simulink model "EVdemo_6"  (R2013b)
settings: Solver=FixedStepDiscrete  SolverMode=SingleTasking  StartTime=0.0  StopTime=650  FixedStep=4e-5  MaxStep=1e-5  RelTol=1e-3
InitFcn:
  | %EV_Param_Update
  | % update the number of strings (discretized)
  | numStrings = round(Opti_numStrings);
  | %disp(['Number of strings: ' num2str(numStrings)])
  | % update the effective capacity based on the number of strings
  | EV_Param.Battery_Det.Rated_Capacity = 28.5*numStrings; %A*hr
  | EV_Param.Battery_Det.DP = 1.5*fliplr([1500 1500 1600 1450 1325 1125 925 675 425 175 ])./8*EV_Param.Battery_Det.Rated_Capacity; % 8 comes from the 8Ahr rated batter data used (normalize and rescale to the rated capacity
  | EV_Param.Battery_Det.CP = fliplr([25 100 200 250 375 550 750 950 1125 1150])./8*EV_Param.Battery_Det.Rated_Capacity;
  | 
  | % update the number of cells in a string (discretized)
  | numSeriesCells = round(Opti_numSeriesCells);
  | %disp(['Number of cells in a string: ' num2str(numSeriesCells)])
  | % update the nominal string volage and charge deficit
  | EV_Param.Battery_Det.Nominal_Voltage = numSeriesCells*cellVolts;
  | BatteryParams(1).Qe_init = 0;%EV_Param.Battery_Det.Rated_Capacity*(1-EV_Param.Battery_Det.Initial_SOC/100); %Ampere*hours
  | 
  | % update the total number of cells, battery pack mass and total vehicle
  | % mass
  | total_cells = numSeriesCells*numStrings;
  | %disp(['Total Number of cells: ' num2str(total_cells)])
  | EV_Param.BatteryMass = BatteryParams(1).cell_mass*total_cells;
  | %disp(['Total Battery Pack Mass: ' num2str(EV_Param.BatteryMass)])
  | EV_Param.Vehicle.Mass = 1300+EV_Param.BatteryMass;
  | 
  | % update the driveline gear ratio
  | EV_Param.Vehicle.Engine_Vehicle_Gear_Ratio = Opti_Vehicle_Gear_Ratio;
  | %disp(['Driveline gear ratio: ' num2str(Opti_Vehicle_Gear_Ratio)])
StartFcn:
  | %tic;
StopFcn:
  | %toc;
  | %disp([Final SOC: ' num2str(SOC_final)])
  | %disp([Final Vehicle Error: ' num2str(normed_SQE_final)])
model workspace (MAT data in the model file):
  SOC_Max_19 = param.Continuous
  SOC_Max_19.Size_ = [1 1]
  SOC_Max_19.Value_ = 68.9908010311
  SOC_Max_19.pID = paramid.Variable
  SOC_Max_19.pID.Name = 'SOC_Max'
  Veh_Err_min_19 = param.Continuous
  Veh_Err_min_19.Size_ = [1 1]
  Veh_Err_min_19.Value_ = 7.40617648417
  Veh_Err_min_19.pID = paramid.Variable
  Veh_Err_min_19.pID.Name = 'Veh_Err_min'
values from neighbouring files (symbols this model uses):
  Drive_Cycle_Num = 8    [startDemo.m]
undefined symbols (not defined in the file or in its folder): Acc_Cmd, BatteryParams, Brake_Set, cell_area, ctrlConst, current_phase_a, Dec_Cmd, direct_current, DiscIntNeverNeededParam, electromagnetic_torque, HEV_Param, Ion, Kt_Temps, Lithium, Mech_Power_kW, Opti_numSeriesCells, Opti_numStrings, Opti_Vehicle_Gear_Ratio, paramVelocityI, paramVelocityP, paramVelocityPICurrentSat, pmsm, quadrature_current, RLoadLoss, rotor_velocity, sigbuilder_block, Ts, Veh_Spd_Ref
libraries: fl_lib x306, nesl_utility x100, LeadAcidBattery_lib x60, simulink x23, powerlib x16, sdl_lib x7, elec_lib x4, electricdrivelib x2, checkpacklib x2, CustomDriveline_lib x2, LiBatteryBlocks x1, Capacitors_lib x1
(part 1 of 7)
Description:
  | Control Velocity of Permanent Magnet Synchronous Machine With Disc Load
  | 
  | Demonstrates a Field-Oriented Control algorithm with Space Vector Modulation for a Permanent Magnet Synchronous Machine (PMSM).
  | The test bench can be used to evaluate the system performance. Examples include turning the motor on, searching for a valid rotor position,
  | transitioning to closed loop operation, and changing speed and torque during closed loop control.
  | The Embedded Processor subsystem contains the controller algorithm (which supports C code generation) as well as simulation models of peripherals.
settings Model: PauseTimes=13.1  SnapshotBufferSize=100  SnapshotInterval=1  CovMetricSettings=dcw  CovHTMLOptions=-sRT=1 -aTS=1 -bRG=1 -bTC=1 -hTR=0 -nFC=0 -scm=1 -bcm=1 -xEv=0  CovModelRefEnable=off  ExtModeTrigDuration=100  Creator=The MathWorks Inc.  LastModifiedBy=rchladny
settings SolverCC: ZeroCrossAlgorithm=Adaptive
settings DataIOCC: LimitDataPoints=off  SaveFormat=StructureWithTime  SaveOutput=off  SaveTime=off  ReturnWorkspaceOutputs=on  StateSaveName=tmp_raccel_xout  SignalLoggingName=SDO_logsout
settings OptimizationCC: InlineParams=on  InlineInvariantSignals=on  EnhancedBackFolding=on  StrengthReduction=on  ExpressionDepthLimit=2147483647  EfficientMapNaN2IntZero=off
settings DebuggingCC: ReadBeforeWriteMsg=DisableAll  WriteAfterWriteMsg=DisableAll  WriteAfterReadMsg=DisableAll  AlgebraicLoopMsg=none  CheckSSInitialOutputMsg=off  MaskedZcDiagnostic=none  IgnoredZcDiagnostic=none  SolverPrmCheckMsg=none  InheritedTsInSrcMsg=none  MultiTaskDSMMsg=none  MultiTaskCondExecSysMsg=none  SingleTaskRateTransMsg=error  IntegerOverflowMsg=none  ParameterPrecisionLossMsg=none  FcnCallInpInsideContextMsg=EnableAllAsWarning  UnconnectedInputMsg=none  UnconnectedOutputMsg=none  UnconnectedLineMsg=none  AssertControl=DisableAll  UnknownTsInhSupMsg=none  StateNameClashWarn=warning
settings HardwareCC: ProdBitPerChar=16  ProdBitPerInt=16  ProdBitPerPointer=16  ProdLargestAtomicInteger=Integer  ProdIntDivRoundTo=Zero  ProdEndianess=LittleEndian  ProdWordSize=16  ProdHWDeviceType=Texas Instruments->C2000  TargetLongLongMode=on  TargetIntDivRoundTo=Zero  TargetEndianess=LittleEndian  TargetHWDeviceType=MATLAB Host  ProdEqTarget=off
settings ModelReferenceCC: UpdateModelReferenceTargets=IfOutOfDate  ModelReferenceNumInstancesAllowed=Single
settings SFSimCC: SFSimEcho=off
settings CodeAppCC: MaxIdLength=128
settings GRTTargetCC: CombineOutputUpdateFcns=off  GRTInterface=on

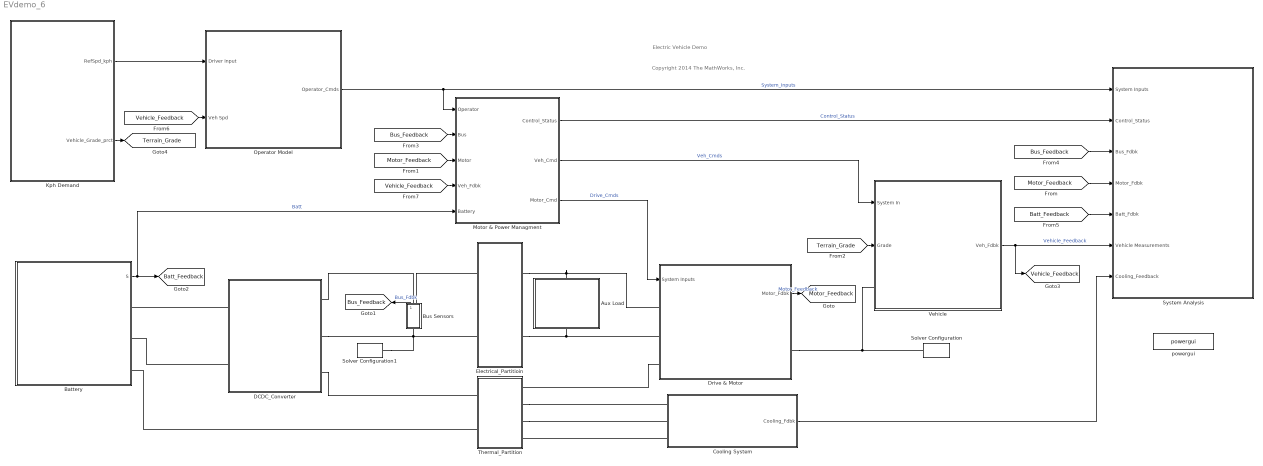
== system EVdemo_6 ==
  note: Electric Vehicle Demo
  note: Copyright 2014 The MathWorks, Inc.
  Aux Load : Subsystem
      mask init:
      | x0=0;%default value
      mask Display: image('auxloads.jpg')
  Battery : Subsystem  Variant=on  OverrideUsingVariant=ETHERM_LUMPED
      settings: AttributesFormatString=%<ActiveVariant>
      mask Display:
      | % Find the active variant
      | ActiveVar = get_param(gcb,'activevariant');
      | % Find the subsystem wrt the active variant
      | blk = find_system(gcbh,'VariantObject',ActiveVar);
      | % Get the Icon
      | ActiveVarCmd = get_param(blk,'MaskDisplay');
      | % Eval
      | eval(ActiveVarCmd);
  Bus Sensors : Subsystem
      mask Display: %image('BNC.jpg')
  Cooling System : Subsystem
      mask Display: image('radiator.jpg')
  DCDC_Converter : Subsystem  Variant=on
      settings: AttributesFormatString=%<ActiveVariant>
      mask Display:
      | % Find the active variant
      | ActiveVar = get_param(gcb,'activevariant');
      | % Find the subsystem wrt the active variant
      | blk = find_system(gcbh,'VariantObject',ActiveVar);
      | % Get the Icon
      | ActiveVarCmd = get_param(blk,'MaskDisplay');
      | % Eval
      | eval(ActiveVarCmd);
      | port_label('RConn',1,'Bus+');
      | port_label('RConn',2,'Bus-');
      | port_label('LConn',1,'Batt+');
      | port_label('LConn',2,'Batt-');
  Drive & Motor : Subsystem  Variant=on  OverrideUsingVariant=SYSYEM_PMSM_CNTRL
      mask Display:
      | % Find the active variant
      | ActiveVar = get_param(gcb,'activevariant');
      | % Find the subsystem wrt the active variant
      | blk = find_system(gcbh,'VariantObject',ActiveVar);
      | % Get the Icon
      | ActiveVarCmd = get_param(blk,'MaskDisplay');
      | % Eval
      | eval(ActiveVarCmd);
  Electrical_Partitioin : Subsystem
  Kph Demand : Subsystem
      mask Display:
      | image('road.JPG')
      | %plotstr=['UrbanCycle' evalin('base','num2str(Drive_Cycle_Num)')];
      | %plot(evalin('base',[plotstr '.time']),evalin('base',[plotstr '.SpdKph']));
      | %text(evalin('base',['0.7*max(' plotstr '.time)']),evalin('base',['0.25*max(' plotstr '.SpdKph)']),evalin('base','num2str(Drive_Cycle_Num)'));
  Motor & Power Managment : Subsystem
      mask Display: image('embedded.jpg')
  Operator Model : Subsystem  Description=""
      mask Display:
      | %fprintf('System\nInputs')
      | image('steering_wheel.jpg')
  Solver Configuration : nesl_utility/Solver Configuration  PhysicalDomain=network_engine_domain  SubClassName=solver  LeftPortType=input  RightPortType=generic  Accelerate=off  Tones=[]  Harmonics=[]  SimulateNoise=off  Profile=off  UseLocalSampling=off  EnableSwitchedLinearOptims=on  FrequencyDomain=off  UseCCode=off  RelTol=0.001  AbsTol=1e-06  MinStep=1e-09  ToWorkspace=off  DoDC=off  ResidualTolerance=1e-8  UseLocalSolver=on  LocalSolverChoice=NE_BACKWARD_EULER_ADVANCER  LocalSolverSampleTime=0.001  DoFixedCost=on  MaxNonlinIter=2  MaxModeIter=2  LinearAlgebra=Sparse  DelaysMemoryBudget=1024
  Solver Configuration1 : nesl_utility/Solver Configuration  PhysicalDomain=network_engine_domain  SubClassName=solver  LeftPortType=input  RightPortType=generic  Accelerate=off  Tones=[]  Harmonics=[]  SimulateNoise=off  Profile=off  UseLocalSampling=off  EnableSwitchedLinearOptims=on  FrequencyDomain=off  UseCCode=off  RelTol=0.001  AbsTol=1e-06  MinStep=1e-09  ToWorkspace=off  DoDC=off  ResidualTolerance=1e-8  UseLocalSolver=on  LocalSolverChoice=NE_BACKWARD_EULER_ADVANCER  LocalSolverSampleTime=0.0002  DoFixedCost=on  MaxNonlinIter=2  MaxModeIter=2  LinearAlgebra=Sparse  DelaysMemoryBudget=1024
  System Analysis : Subsystem  Description=|
      | System Analysis for Speed Control Design
      | 
      | Analyize and plot signals used to analyize performance of
      | speed  control designs
      mask Display:
      | %fprintf('System\nAnalysis')
      | image('dashboard_2.jpg')
  Thermal_Partition : Subsystem
  Vehicle : Subsystem  Variant=on  OverrideUsingVariant=DETAILED_VEHICLE
      settings: AttributesFormatString=%<ActiveVariant>
      mask Display:
      | % Find the active variant
      | ActiveVar = get_param(gcb,'activevariant');
      | % Find the subsystem wrt the active variant
      | blk = find_system(gcbh,'VariantObject',ActiveVar);
      | % Get the Icon
      | ActiveVarCmd = get_param(blk,'MaskDisplay');
      | % Eval
      | eval(ActiveVarCmd);
  powergui : powerlib/powergui  Priority=1  SimulationMode=Continuous  SolverType=Tustin  SampleTime=50e-6  frequency=60  SPID=on  DisableSnubberDevices=off  DisableRonSwitches=off  DisableVfSwitches=off  SwTol=0  Interpol=off  DisplayEquations=off  frequencyindice=0  Pbase=100e6  ErrMax=1e-4  Iterations=50  UnitsV=kV  UnitsW=MW  FunctionMessages=off  echomessages=off  HookPort=off  EnableUseOfTLC=off  x0status=blocks  RestoreLinks=warning  ResistiveCurrentMeasurement=off  Frange=[0:2:500]  Ylog=off  Xlog=on  ShowGrid=off  save=off  variable=ZData  ZoomFFT=off  StartTime=0.0  cycles=1  DisplayStyle=1  fundamental=60  FreqAxis=off  MaxFrequency=1000  frequencyindicesteady=1  RmsSteady=1  display=off  Ts=0  methode=off
  tag scope: Batt_Feedback=global, Bus_Feedback=global, Motor_Feedback=global, Terrain_Grade=global, Vehicle_Feedback=global
  wires:
  Operator Model/1(Operator_Cmds) -> Motor & Power Managment/1(Operator), System Analysis/1(System Inputs)  "System_Inputs"
  Drive & Motor/1(Motor_Fdbk) -> [Motor_Feedback]  "Motor_Feedback"
  [Motor_Feedback] -> System Analysis/4(Motor_Fdbk)
  Vehicle/1(Veh_Fdbk) -> [Vehicle_Feedback], System Analysis/6(Vehicle Measurements)  "Vehicle_Feedback"
  Bus Sensors/1(Output) -> [Bus_Feedback]  "Bus_Fdbk"
  Battery/1(S) -> [Batt_Feedback], Motor & Power Managment/5(Battery)  "Batt"
  Motor & Power Managment/2(Veh_Cmd) -> Vehicle/1(System In)  "Veh_Cmds"
  [Motor_Feedback] -> Motor & Power Managment/3(Motor)
  [Bus_Feedback] -> Motor & Power Managment/2(Bus)
  Motor & Power Managment/1(Control_Status) -> System Analysis/2(Control_Status)  "Control_Status"
  Motor & Power Managment/3(Motor_Cmd) -> Drive & Motor/1(System Inputs)  "Drive_Cmds"
  [Vehicle_Feedback] -> Operator Model/2(Veh Spd)
  [Bus_Feedback] -> System Analysis/3(Bus_Fdbk)
  [Batt_Feedback] -> System Analysis/5(Batt_Fdbk)
  Kph Demand/1(RefSpd_kph) -> Operator Model/1(Driver Input)
  Kph Demand/2(Vehicle_Grade_prct) -> [Terrain_Grade]
  [Terrain_Grade] -> Vehicle/2(Grade)
  Cooling System/1(Cooling_Fdbk) -> System Analysis/7(Cooling_Feedback)
  [Vehicle_Feedback] -> Motor & Power Managment/4(Veh_Fdbk)
  connections:
  DCDC_Converter/LConn2 -- Battery/RConn2
  DCDC_Converter/LConn1 -- Battery/RConn1
  Aux Load/RConn1 -- Drive & Motor/LConn1 -- Electrical_Partitioin/RConn1
  Bus Sensors/RConn1 -- DCDC_Converter/RConn1
  Drive & Motor/RConn1 -- Solver Configuration/RConn1 -- Vehicle/LConn1
  Aux Load/LConn1 -- Drive & Motor/LConn2 -- Electrical_Partitioin/RConn2
  Solver Configuration1/RConn1 -- DCDC_Converter/RConn2 -- Bus Sensors/LConn1 -- Electrical_Partitioin/LConn2
  Bus Sensors/RConn2 -- Electrical_Partitioin/LConn1
  Thermal_Partition/LConn2 -- Battery/RConn3
  DCDC_Converter/RConn3 -- Thermal_Partition/LConn1
  Drive & Motor/LConn3 -- Thermal_Partition/RConn1
  Thermal_Partition/RConn2 -- Cooling System/LConn1
  Thermal_Partition/RConn3 -- Cooling System/LConn2
  Cooling System/LConn3 -- Thermal_Partition/RConn4

== system EVdemo_6/Aux Load ==
  2kw Accessory Load : Step  After=2e3
  Controlled Current Source : fl_lib/Electrical/Electrical Sources/Controlled Current Source  i_Log=off  v_Log=off  LocalVarNames=|i|v  LocalVarDescs=|i|v  LocalVarLogging=[0 0]
  Divide : Product  Inputs=*/
  Min V : Constant  Value=20  SampleTime=-1
  MinMax : MinMax  Function=max  Inputs=2
  Off : Constant  Value=0  SampleTime=-1
  PS-Simulink Converter : nesl_utility/PS-Simulink Converter  PhysicalDomain=network_engine_domain  SubClassName=ps_output  LeftPortType=input  RightPortType=output  PseudoPeriodic=off  Frequencies=[]  Unit=1  AffineConversion=off
  Rate Limiter : RateLimiter  RisingSlewLimit=1e3  FallingSlewLimit=-1e3  SampleTimeMode=inherited
  Simulink-PS Converter : nesl_utility/Simulink-PS Converter  PhysicalDomain=network_engine_domain  SubClassName=ps_input  LeftPortType=input  RightPortType=output  PseudoPeriodic=off  Frequencies=[]  NoiseDistribution=none  NoiseParameters=[]  Unit=1  AffineConversion=off  InputFiltering=off  SimscapeFilterOrder=1  InputFilterTimeConstant=0.001  UdotUserProvided=1
  Switch : Switch  Criteria=u2 > Threshold  Threshold=20
  Unit Delay : UnitDelay  SampleTime=-1
  Voltage Sensor : fl_lib/Electrical/Electrical Sensors/Voltage Sensor  i1_Log=off  v1_Log=off  LocalVarNames=|i1|v1  LocalVarDescs=|i1|v1  LocalVarLogging=[0 0]
  + : PMIOPort  Port=1  Side=Right
  - : PMIOPort  Port=2  Side=Left
  wires:
  PS-Simulink Converter/1 -> Switch/2, MinMax/1
  Divide/1 -> Unit Delay/1
  MinMax/1 -> Divide/2
  Min V/1 -> MinMax/2
  Unit Delay/1 -> Simulink-PS Converter/1
  Off/1 -> Switch/3
  Switch/1 -> Divide/1
  2kw Accessory Load/1 -> Rate Limiter/1
  Rate Limiter/1 -> Switch/1
  connections:
  Voltage Sensor/RConn2 -- Controlled Current Source/LConn1 -- -/RConn1
  Voltage Sensor/LConn1 -- Controlled Current Source/RConn2 -- +/RConn1
  PS-Simulink Converter/LConn1 -- Voltage Sensor/RConn1
  Controlled Current Source/RConn1 -- Simulink-PS Converter/RConn1

== system EVdemo_6/Battery ==
  Cells : Subsystem  VariantControl=CELLS_BATT
      mask Display:
      | image(imread('HEV_Battery_Cells_IMAGE.jpg'));
      | port_label('RConn',1,'+');
      | port_label('RConn',2,'-');
      | port_label('RConn',3,'H')
      | port_label('output',1,'S');
  Electro-Thermal : Subsystem  VariantControl=ETHERM_LUMPED
      mask Display:
      | image(imread('battery.jpg'));
      | port_label('RConn',1,'+')
      | port_label('RConn',2,'-')
      | port_label('RConn',3,'H')
      | port_label('output',1,'S');
  Generic : Subsystem  VariantControl=GENERIC_1_BATT
      mask Display:
      | image(imread('HEV_Battery_Custom_IMAGE.jpg'));
      | port_label('RConn',1,'+');
      | port_label('RConn',2,'-');
      | port_label('RConn',3,'H')
      | port_label('output',1,'S');
  Generic1 : Subsystem  VariantControl=GENERIC_2_BATT
      mask Display:
      | image(imread('HEV_Battery_Generic_IMAGE.jpg'));
      | port_label('RConn',1,'+');
      | port_label('RConn',2,'-');
      | port_label('RConn',3,'H')
      | port_label('output',1,'S');
  Predefined : Subsystem  VariantControl=PREDEF_BATT
      mask Display:
      | image(imread('HEV_Battery_Detailed_IMAGE.jpg'));
      | port_label('RConn',1,'+');
      | port_label('RConn',2,'-');
      | port_label('RConn',3,'H')
      | port_label('output',1,'S');
  RCGeneric : Subsystem  VariantControl=GENERIC_RC_BATT
      mask Display:
      | image(imread('HEV_Battery_GenericRC_IMAGE.jpg'));
      | port_label('RConn',1,'+');
      | port_label('RConn',2,'-');
      | port_label('RConn',3,'H')
      | port_label('output',1,'S');
  + : PMIOPort  Port=1  Side=Right
  - : PMIOPort  Port=2  Side=Right
  H : PMIOPort  Tag=PMCPort  Port=3  Side=Right
  S : Outport

== system EVdemo_6/Bus Sensors ==
  Bus Creator : BusCreator  Inputs=3
  Current Sensor : fl_lib/Electrical/Electrical Sensors/Current Sensor  i1_Log=off  v1_Log=off  LocalVarNames=|i1|v1  LocalVarDescs=|i1|v1  LocalVarLogging=[0 0]
  Gain : Gain  Gain=1e-3
  LPF : Subsystem  mask{w=2*pi*250}
      mask prompts: w "w(rad/s)"
      mask Display:
      | fprintf('LPF')
      | port_label('output', 1, 'out')
      | port_label('input', 1, 'in')
  LPF1 : Subsystem  mask{w=2*pi*250}
      mask prompts: w "w(rad/s)"
      mask Display:
      | fprintf('LPF')
      | port_label('output', 1, 'out')
      | port_label('input', 1, 'in')
  PS-Simulink Converter : nesl_utility/PS-Simulink Converter  PhysicalDomain=network_engine_domain  SubClassName=ps_output  LeftPortType=input  RightPortType=output  PseudoPeriodic=off  Frequencies=[]  Unit=1  AffineConversion=off
  PS-Simulink Converter1 : nesl_utility/PS-Simulink Converter  PhysicalDomain=network_engine_domain  SubClassName=ps_output  LeftPortType=input  RightPortType=output  PseudoPeriodic=off  Frequencies=[]  Unit=1  AffineConversion=off
  Product : Product
  Voltage Sensor : fl_lib/Electrical/Electrical Sensors/Voltage Sensor  i1_Log=off  v1_Log=off  LocalVarNames=|i1|v1  LocalVarDescs=|i1|v1  LocalVarLogging=[0 0]
  +in : PMIOPort  Port=1  Side=Right
  - : PMIOPort  Port=2  Side=Left
  +out : PMIOPort  Port=3  Side=Right
  Output : Outport
  wires:
  Gain/1 -> Bus Creator/3  "Bus_Power_kW"
  Product/1 -> Gain/1
  PS-Simulink Converter/1 -> LPF/1(In)
  PS-Simulink Converter1/1 -> LPF1/1(In)
  LPF/1(Out) -> Bus Creator/2, Product/2  "Voltage"
  LPF1/1(Out) -> Bus Creator/1, Product/1  "Current"
  Bus Creator/1 -> Output/1  "Bus_System"
  connections:
  Current Sensor/LConn1 -- +in/RConn1 -- Voltage Sensor/LConn1
  Voltage Sensor/RConn2 -- -/RConn1
  Voltage Sensor/RConn1 -- PS-Simulink Converter/LConn1
  Current Sensor/RConn1 -- PS-Simulink Converter1/LConn1
  +out/RConn1 -- Current Sensor/RConn2

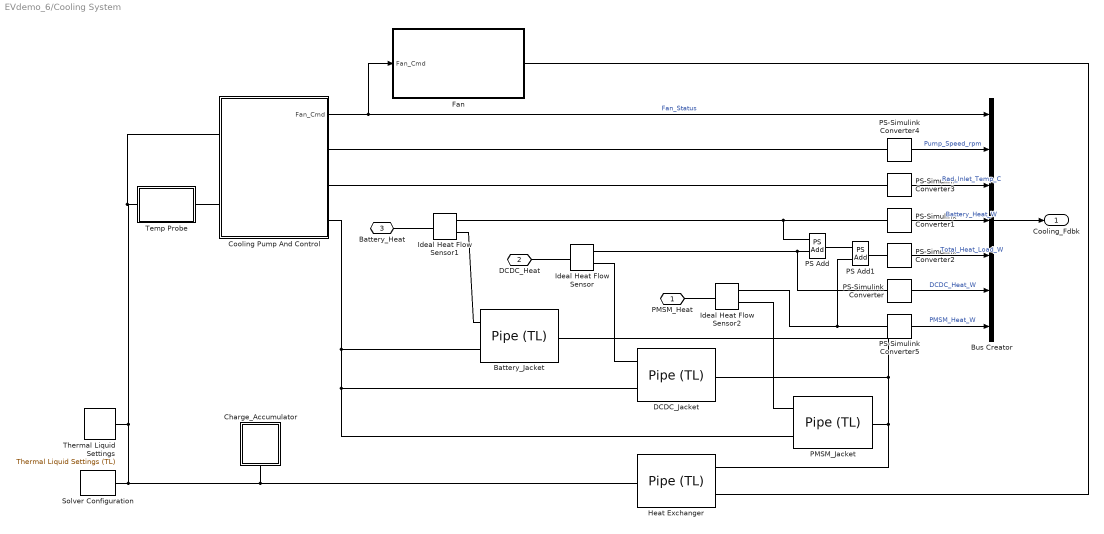
== system EVdemo_6/Cooling System ==
  Battery_Jacket : fl_lib/Thermal Liquid/Elements/Pipe (TL)  dynamic_compressibility=0  inertia=0  length=.75 m  length_add=1 m  Dh=4*(.01*.015)/(.015+2*.01) m  area=.01*.015 m^2  shape_factor=.01/.04*64  roughness=1.5e-5 m  Re_l=2e+3  Re_t=4e+3  Nu_coeff_l=[ 1.86 0.33 0.33 0.33 0.14 ]  Nu_coeff_t=[ 0.023 0.8 0.33 0 0 ]  T0=BatteryParams(1).T_init K  p0=1 atm  mdot0=0.1 kg/s  LocalVarLogging=[]
  Bus Creator : BusCreator  Inputs=7
  Charge_Accumulator : Subsystem
  Cooling Pump And Control : Subsystem
  DCDC_Jacket : fl_lib/Thermal Liquid/Elements/Pipe (TL)  dynamic_compressibility=0  inertia=0  length=.3 m  length_add=1 m  Dh=4*(.01*.04)/(.04+2*.01) m  area=.01*.04 m^2  shape_factor=.01/.04*64  roughness=1.5e-5 m  Re_l=2e+3  Re_t=4e+3  Nu_coeff_l=[ 1.86 0.33 0.33 0.33 0.14 ]  Nu_coeff_t=[ 0.023 0.8 0.33 0 0 ]  T0=BatteryParams(1).T_init K  p0=1 atm  mdot0=0.1 kg/s  LocalVarLogging=[]
  Fan : Subsystem
  Heat Exchanger : fl_lib/Thermal Liquid/Elements/Pipe (TL)  dynamic_compressibility=0  inertia=0  length=1.5 m  length_add=1 m  Dh=.03 m  area=pi/4*.03^2 m^2  shape_factor=64  roughness=1.5e-5 m  Re_l=2e+3  Re_t=4e+3  Nu_coeff_l=[ 1.86 0.33 0.33 0.33 0.14 ]  Nu_coeff_t=[ 0.023 0.8 0.33 0 0 ]  T0=BatteryParams(1).T_init K  p0=1 atm  mdot0=0.1 kg/s  LocalVarLogging=[]
  Ideal Heat Flow Sensor : fl_lib/Thermal/Thermal Sensors/Ideal Heat Flow Sensor  Q_Log=off  T_Log=off  LocalVarNames=|Q|T  LocalVarDescs=|Q|T  LocalVarLogging=[0 0]
  Ideal Heat Flow Sensor1 : fl_lib/Thermal/Thermal Sensors/Ideal Heat Flow Sensor  Q_Log=off  T_Log=off  LocalVarNames=|Q|T  LocalVarDescs=|Q|T  LocalVarLogging=[0 0]
  Ideal Heat Flow Sensor2 : fl_lib/Thermal/Thermal Sensors/Ideal Heat Flow Sensor  Q_Log=off  T_Log=off  LocalVarNames=|Q|T  LocalVarDescs=|Q|T  LocalVarLogging=[0 0]
  PMSM_Jacket : fl_lib/Thermal Liquid/Elements/Pipe (TL)  dynamic_compressibility=0  inertia=0  length=.3 m  length_add=1 m  Dh=4*(.01*.04)/(.04+2*.01) m  area=.01*.04 m^2  shape_factor=.01/.04*64  roughness=1.5e-5 m  Re_l=2e+3  Re_t=4e+3  Nu_coeff_l=[ 1.86 0.33 0.33 0.33 0.14 ]  Nu_coeff_t=[ 0.023 0.8 0.33 0 0 ]  T0=BatteryParams(1).T_init K  p0=1 atm  mdot0=0.1 kg/s  LocalVarLogging=[]
  PS Add : fl_lib/Physical Signals/Functions/PS Add  LocalVarLogging=[]
  PS Add1 : fl_lib/Physical Signals/Functions/PS Add  LocalVarLogging=[]
  PS-Simulink Converter{,1..2,4..5} (5 alike) : nesl_utility/PS-Simulink Converter  PhysicalDomain=network_engine_domain  SubClassName=ps_output  LeftPortType=input  RightPortType=output  PseudoPeriodic=off  Frequencies=[]  Unit=1  AffineConversion=off
  PS-Simulink Converter3 : nesl_utility/PS-Simulink Converter  PhysicalDomain=network_engine_domain  SubClassName=ps_output  LeftPortType=input  RightPortType=output  PseudoPeriodic=off  Frequencies=[]  Unit=C  AffineConversion=off
  Solver Configuration : nesl_utility/Solver Configuration  PhysicalDomain=network_engine_domain  SubClassName=solver  LeftPortType=input  RightPortType=generic  Accelerate=off  Tones=[]  Harmonics=[]  SimulateNoise=off  Profile=off  UseLocalSampling=off  EnableSwitchedLinearOptims=on  FrequencyDomain=off  UseCCode=off  RelTol=0.001  AbsTol=1e-06  MinStep=1e-09  ToWorkspace=off  DoDC=off  ResidualTolerance=1e-09  UseLocalSolver=on  LocalSolverChoice=NE_BACKWARD_EULER_ADVANCER  LocalSolverSampleTime=0.1  DoFixedCost=on  MaxNonlinIter=2  MaxModeIter=2  LinearAlgebra=Sparse  DelaysMemoryBudget=1024
  Temp Probe : Subsystem
  Thermal Liquid Settings : fl_lib/Thermal Liquid/Utilities/Thermal Liquid Settings (TL)  pT_region_flag=0  T_min=273.16 K  T_max=373.16 K  p_min=0.1 bar  p_max=500 bar  T_TLU=[273.1600 : 10 : 373.16]' K  p_TLU=[0.1, 1, 50 : 50 : 500] bar  pT_validity_TLU=ones(11, 12)  rho_TLU=[999.8, 999.8, 1002.3, 1004.8, 1007.3, 1009.7, 1012.2, 1014.5, 1016.9, 1019.2, 1021.5, 1023.8; 999.7, 999.7, 1002.0, 1004.4, 1006.7, 1009.0, 1011.3, 1013.5, 1015.8, 1018.0, 1020.2, 1022.3; 998.2, 998.2, 1000.4, 1002.7, 1004.9, 1007.1, 1009.3, 1011.5, 1013.6, 1015.7, 1017.8, 1019.9; 995.6, 995.6, 997.8, 1000.0, 1002.2, 1004.3, 1006.5, 1008.6, 1010.7, 1012.7, 1014.8, 1016.8; 992.2, 992.2, 994.4, 996.5, 998.6, 1000.8, 1002.9, 1004.9, 1007.0, 1009.0, 1011.0, 1013.0; 988.0, 988.0, 990.2, 992.3, 994.4, 996.5, 998.6, 1000.7, 1002.7, 1004.7, 1006.7, 1008.7; 983.2, 983.2, 985.3, 987.5, 989.6, 991.7, 993.8, 995.8, 997.9, 999.9, 1001.9, 1003.9; 977.8, 977.8, 979.9, 982.1, 984.2, 986.3, 988.4, 990.5, 992.5, 994.6, 996.6, 998.6; 971.8, 971.8, 974.0, 976.2, 978.3, 980.5, 982.6, 984.7, 986.8, 988.8, 990.9, 992.9; 965.3, 965.3, 967.5, 969.8, 972.0, 974.2, 976.3, 978.5, 980.6, 982.7, 984.7, 986.8; 958.8, 958.8, 960.6, 962.9, 965.2, 967.4, 969.6, 971.8, 974.0, 976.1, 978.2, 980.3] kg/m^3  u_TLU=[0.0002, 0.0018, 0.0860, 0.1588, 0.2190, 0.2670, 0.3034, 0.3288, 0.3436, 0.3483, 0.3435, 0.3294; 42.0620, 42.0600, 41.9350, 41.8040, 41.6680, 41.5270, 41.3820, 41.2330, 41.0810, 40.9240, 40.7630, 40.5990; 83.9530, 83.9480, 83.6510, 83.3490, 83.0490, 82.7490, 82.4510, 82.1530, 81.8560, 81.5600, 81.2650, 80.9710; 125.7700, 125.7600, 125.3100, 124.8600, 124.4100, 123.9700, 123.5300, 123.1000, 122.6800, 122.2500, 121.8400, 121.4200; 167.5700, 167.5600, 166.9600, 166.3700, 165.7900, 165.2100, 164.6500, 164.0900, 163.5400, 163.0000, 162.4600, 161.9400; 209.3600, 209.3600, 208.6300, 207.9000, 207.1900, 206.4800, 205.7900, 205.1100, 204.4500, 203.7900, 203.1400, 202.5000; 251.1900, 251.1900, 250.3300, 249.4700, 248.6200, 247.7900, 246.9800, 246.1800, 245.3900, 244.6200, 243.8600, 243.1200; 293.0600, 293.0600, 292.0700, 291.0700, 290.1000, 289.1400, 288.2000, 287.2800, 286.3800, 285.4900, 284.6200, 283.7700; 334.9900, 334.9900, 333.8600, 332.7300, 331.6300, 330.5400, 329.4800, 328.4400, 327.4100, 326.4100, 325.4300, 324.4600; 377.0000, 377.0000, 375.7300, 374.4600, 373.2200, 372.0000, 370.8100, 369.6400, 368.5000, 367.3800, 366.2700, 365.1900; 419.0100, 419.0100, 417.6900, 416.2700, 414.8900, 413.5400, 412.2100, 410.9100, 409.6400, 408.4000, 407.1700, 405.9800] J/g  nu_TLU=[1.7917, 1.7914, 1.7763, 1.7615, 1.7473, 1.7338, 1.7208, 1.7085, 1.6967, 1.6854, 1.6747, 1.6645; 1.3061, 1.3059, 1.2986, 1.2914, 1.2845, 1.2779, 1.2716, 1.2656, 1.2598, 1.2543, 1.2491, 1.2441; 1.0032, 1.0032, 0.9995, 0.9959, 0.9924, 0.9891, 0.9859, 0.9829, 0.9801, 0.9774, 0.9748, 0.9724; 0.8006, 0.8005, 0.7987, 0.7970, 0.7953, 0.7937, 0.7922, 0.7908, 0.7894, 0.7881, 0.7870, 0.7859; 0.6577, 0.6577, 0.6570, 0.6562, 0.6555, 0.6548, 0.6543, 0.6537, 0.6532, 0.6528, 0.6523, 0.6520; 0.5530, 0.5530, 0.5529, 0.5527, 0.5526, 0.5525, 0.5524, 0.5524, 0.5524, 0.5524, 0.5524, 0.5525; 0.4739, 0.4739, 0.4741, 0.4743, 0.4745, 0.4747, 0.4750, 0.4753, 0.4755, 0.4758, 0.4762, 0.4765; 0.4127, 0.4127, 0.4131, 0.4135, 0.4139, 0.4143, 0.4148, 0.4152, 0.4157, 0.4162, 0.4167, 0.4172; 0.3643, 0.3643, 0.3648, 0.3654, 0.3659, 0.3665, 0.3670, 0.3676, 0.3682, 0.3688, 0.3694, 0.3700; 0.3254, 0.3254, 0.3261, 0.3267, 0.3273, 0.3280, 0.3286, 0.3293, 0.3299, 0.3306, 0.3312, 0.3319; 0.2866, 0.2866, 0.2945, 0.2952, 0.2959, 0.2965, 0.2972, 0.2979, 0.2986, 0.2993, 0.3000, 0.3007] mm^2/s  cp_TLU=[4.2199, 4.2194, 4.1957, 4.1726, 4.1508, 4.1300, 4.1103, 4.0916, 4.0738, 4.0569, 4.0408, 4.0254; 4.1955, 4.1951, 4.1769, 4.1592, 4.1422, 4.1259, 4.1103, 4.0954, 4.0812, 4.0676, 4.0545, 4.0421; 4.1843, 4.1840, 4.1690, 4.1543, 4.1401, 4.1264, 4.1133, 4.1007, 4.0885, 4.0768, 4.0656, 4.0548; 4.1801, 4.1798, 4.1667, 4.1538, 4.1413, 4.1293, 4.1177, 4.1064, 4.0956, 4.0851, 4.0750, 4.0653; 4.1796, 4.1794, 4.1675, 4.1558, 4.1444, 4.1334, 4.1227, 4.1123, 4.1023, 4.0926, 4.0832, 4.0741; 4.1813, 4.1813, 4.1702, 4.1592, 4.1484, 4.1380, 4.1279, 4.1181, 4.1086, 4.0993, 4.0903, 4.0816; 4.1850, 4.1850, 4.1742, 4.1636, 4.1532, 4.1432, 4.1334, 4.1239, 4.1146, 4.1056, 4.0969, 4.0884; 4.1901, 4.1901, 4.1795, 4.1690, 4.1588, 4.1489, 4.1393, 4.1299, 4.1207, 4.1118, 4.1032, 4.0947; 4.1968, 4.1968, 4.1862, 4.1757, 4.1655, 4.1555, 4.1458, 4.1364, 4.1273, 4.1183, 4.1096, 4.1012; 4.2052, 4.2052, 4.1944, 4.1837, 4.1733, 4.1632, 4.1534, 4.1438, 4.1345, 4.1255, 4.1166, 4.1080; 4.2136, 4.2136, 4.2045, 4.1935, 4.1828, 4.1724, 4.1623, 4.1524, 4.1429, 4.1335, 4.1245, 4.1157] J/K/g  k_TLU=[561.0400, 561.0900, 563.8000, 566.5600, 569.3200, 572.0800, 574.8200, 577.5400, 580.2400, 582.9200, 585.5700, 588.1800; 580.0200, 580.0700, 582.4500, 584.8800, 587.3200, 589.7500, 592.1800, 594.6100, 597.0200, 599.4200, 601.8000, 604.1600; 598.4400, 598.4800, 600.7300, 603.0300, 605.3300, 607.6400, 609.9400, 612.2400, 614.5400, 616.8200, 619.1000, 621.3600; 615.4800, 615.5200, 617.7300, 620.0000, 622.2600, 624.5400, 626.8100, 629.0700, 631.3400, 633.6000, 635.8500, 638.0900; 630.6000, 630.6400, 632.8700, 635.1500, 637.4400, 639.7200, 642.0100, 644.2900, 646.5700, 648.8400, 651.1100, 653.3600; 643.6100, 643.6100, 645.8800, 648.2100, 650.5300, 652.8600, 655.1800, 657.5100, 659.8200, 662.1400, 664.4400, 666.7400; 654.3900, 654.3900, 656.7300, 659.1200, 661.5000, 663.8900, 666.2700, 668.6500, 671.0200, 673.3800, 675.7400, 678.0900; 663.1300, 663.1300, 665.5400, 668.0000, 670.4600, 672.9100, 675.3600, 677.8000, 680.2400, 682.6700, 685.0900, 687.5000; 670.0200, 670.0200, 672.5100, 675.0500, 677.5900, 680.1200, 682.6400, 685.1600, 687.6700, 690.1700, 692.6600, 695.1400; 675.2700, 675.2700, 677.8500, 680.4800, 683.1100, 685.7300, 688.3400, 690.9400, 693.5300, 696.1100, 698.6800, 701.2400; 680.5200, 680.5200, 681.7700, 684.5000, 687.2200, 689.9400, 692.6400, 695.3400, 698.0200, 700.6900, 703.3500, 706.0000] mW/m/K  beta_TLU=[1.9649, 1.9654, 1.9929, 2.0213, 2.0499, 2.0787, 2.1078, 2.1372, 2.1668, 2.1966, 2.2268, 2.2572; 2.0913, 2.0918, 2.1191, 2.1471, 2.1752, 2.2036, 2.2322, 2.2610, 2.2899, 2.3191, 2.3485, 2.3781; 2.1786, 2.1791, 2.2067, 2.2350, 2.2634, 2.2919, 2.3206, 2.3494, 2.3784, 2.4075, 2.4367, 2.4661; 2.2332, 2.2337, 2.2619, 2.2908, 2.3197, 2.3487, 2.3778, 2.4070, 2.4363, 2.4657, 2.4951, 2.5246; 2.2600, 2.2605, 2.2895, 2.3191, 2.3487, 2.3784, 2.4081, 2.4378, 2.4675, 2.4973, 2.5272, 2.5571; 2.2638, 2.2638, 2.2936, 2.3240, 2.3544, 2.3848, 2.4151, 2.4455, 2.4758, 2.5062, 2.5365, 2.5669; 2.2472, 2.2472, 2.2779, 2.3092, 2.3403, 2.3715, 2.4025, 2.4336, 2.4646, 2.4955, 2.5264, 2.5573; 2.2140, 2.2140, 2.2455, 2.2776, 2.3096, 2.3415, 2.3733, 2.4050, 2.4367, 2.4683, 2.4998, 2.5313; 2.1668, 2.1668, 2.1992, 2.2321, 2.2649, 2.2976, 2.3301, 2.3626, 2.3949, 2.4272, 2.4593, 2.4914; 2.1081, 2.1081, 2.1413, 2.1750, 2.2086, 2.2421, 2.2754, 2.3085, 2.3415, 2.3744, 2.4072, 2.4399; 2.0494, 2.0494, 2.0739, 2.1084, 2.1428, 2.1770, 2.2110, 2.2449, 2.2786, 2.3121, 2.3455, 2.3788] GPa  alpha_TLU=1e-4 * [0.6790, 0.6760, 0.4900, 0.3070, 0.1300, - 0.0410, - 0.2060, - 0.3650, - 0.5190, - 0.6680, - 0.8110, - 0.9490; - 0.8780, - 0.8810, - 0.9980, - 1.1140, - 1.2270, - 1.3370, - 1.4450, - 1.5490, - 1.6510, - 1.7500, - 1.8460, - 1.9390; - 2.0680, - 2.0690, - 2.1410, - 2.2130, - 2.2830, - 2.3520, - 2.4200, - 2.4860, - 2.5510, - 2.6140, - 2.6760, - 2.7360; - 3.0340, - 3.0350, - 3.0740, - 3.1130, - 3.1520, - 3.1910, - 3.2290, - 3.2670, - 3.3050, - 3.3410, - 3.3770, - 3.4130; - 3.8550, - 3.8560, - 3.8700, - 3.8840, - 3.8990, - 3.9140, - 3.9300, - 3.9460, - 3.9610, - 3.9770, - 3.9930, - 4.0090; - 4.5780, - 4.5780, - 4.5720, - 4.5660, - 4.5620, - 4.5580, - 4.5550, - 4.5520, - 4.5500, - 4.5490, - 4.5480, - 4.5470; - 5.2330, - 5.2330, - 5.2090, - 5.1860, - 5.1650, - 5.1440, - 5.1250, - 5.1070, - 5.0900, - 5.0740, - 5.0590, - 5.0450; - 5.8400, - 5.8400, - 5.8010, - 5.7620, - 5.7250, - 5.6910, - 5.6570, - 5.6250, - 5.5950, - 5.5660, - 5.5380, - 5.5120; - 6.4140, - 6.4140, - 6.3600, - 6.3070, - 6.2560, - 6.2080, - 6.1610, - 6.1170, - 6.0740, - 6.0330, - 5.9940, - 5.9560; - 6.9670, - 6.9670, - 6.8980, - 6.8310, - 6.7660, - 6.7050, - 6.6460, - 6.5890, - 6.5350, - 6.4820, - 6.4320, - 6.3840; - 7.5190, - 7.5190, - 7.4230, - 7.3420, - 7.2640, - 7.1890, - 7.1180, - 7.0490, - 6.9830, - 6.9200, - 6.8590, - 6.8000] 1/K  G_min=1e-3 W/K  p_atm=1 atm  LocalVarLogging=[]
  PMSM_Heat : PMIOPort  Port=1  Side=Left
  DCDC_Heat : PMIOPort  Port=2  Side=Left
  Battery_Heat : PMIOPort  Port=3  Side=Left
  Cooling_Fdbk : Outport
  wires:
  PS-Simulink Converter/1 -> Bus Creator/6  "DCDC_Heat_W"
  PS-Simulink Converter2/1 -> Bus Creator/5  "Total_Heat_Load_W"
  PS-Simulink Converter1/1 -> Bus Creator/4  "Battery_Heat_W"
  PS-Simulink Converter3/1 -> Bus Creator/3  "Rad_Inlet_Temp_C"
  PS-Simulink Converter4/1 -> Bus Creator/2  "Pump_Speed_rpm"
  Cooling Pump And Control/1(Fan_Cmd) -> Fan/1(Fan_Cmd), Bus Creator/1  "Fan_Status"
  Bus Creator/1 -> Cooling_Fdbk/1
  PS-Simulink Converter5/1 -> Bus Creator/7  "PMSM_Heat_W"
  connections:
  Ideal Heat Flow Sensor/RConn1 -- PS-Simulink Converter/LConn1 -- PS Add/LConn2
  Cooling Pump And Control/LConn1 -- Temp Probe/RConn1 -- Solver Configuration/RConn1 -- Heat Exchanger/RConn1 -- Charge_Accumulator/LConn1 -- Thermal Liquid Settings/RConn1
  DCDC_Jacket/RConn1 -- Battery_Jacket/RConn1 -- Heat Exchanger/LConn1 -- PMSM_Jacket/RConn1
  Temp Probe/LConn1 -- Cooling Pump And Control/LConn2
  PS-Simulink Converter3/LConn1 -- Cooling Pump And Control/RConn2
  Ideal Heat Flow Sensor/RConn2 -- DCDC_Jacket/LConn2
  Ideal Heat Flow Sensor1/RConn2 -- Battery_Jacket/LConn2
  Cooling Pump And Control/RConn3 -- Battery_Jacket/LConn1 -- PMSM_Jacket/LConn1 -- DCDC_Jacket/LConn1
  Ideal Heat Flow Sensor1/RConn1 -- PS Add/LConn1 -- PS-Simulink Converter1/LConn1
  DCDC_Heat/RConn1 -- Ideal Heat Flow Sensor/LConn1
  Battery_Heat/RConn1 -- Ideal Heat Flow Sensor1/LConn1
  Cooling Pump And Control/RConn1 -- PS-Simulink Converter4/LConn1
  Fan/RConn1 -- Heat Exchanger/LConn2
  PMSM_Heat/RConn1 -- Ideal Heat Flow Sensor2/LConn1
  Ideal Heat Flow Sensor2/RConn1 -- PS Add1/LConn2 -- PS-Simulink Converter5/LConn1
  PS Add/RConn1 -- PS Add1/LConn1
  PS Add1/RConn1 -- PS-Simulink Converter2/LConn1
  Ideal Heat Flow Sensor2/RConn2 -- PMSM_Jacket/LConn2

== system EVdemo_6/DCDC_Converter ==
  note: 1) Only subsystems can be added as variant choices at this level
      | 2) Blocks cannot be connected at this level as connectivity is
      | automatically determined at simulation, based on the active variant
  Detailed DC/DC Converter : Subsystem  VariantControl=DETALIED_VEHICLE
      mask init:
      | [X1,X1m,X2,X2m,X3,X4,Y1,Y1m,Y2,Y2m,Y3,Y4,color1,color2]=spsdrivelogo;
      mask Display:
      | image(imread('HEV_DCDC_Switching_IMAGE.jpg'));
      | port_label('RConn',1,'Bus+');
      | port_label('RConn',2,'Bus-');
      | port_label('LConn',1,'Batt+');
      | port_label('LConn',2,'Batt-');
      | port_label('RConn',3,'H');
      | text(0.05,0.5,'In');
      | text(0.85,0.5,'Out');
  System DC-DC Converter : Subsystem  VariantControl=SYSTEM_DCDC  mask{Vout=EV_Param.DCDCConv.Output_Voltage, RLoadLoss=EV_Param.DCDCConv.Resistance_Losses, Kp=EV_Param.DCDCConv.Kp, Ki=EV_Param.DCDCConv.Ki}
      mask prompts: Vout "Output Voltage (V)"; RLoadLoss "Resistance, Load Dependent Losses (Ohm)"; Kp "Proportional Gain"; Ki "Integral Gain"
      mask Display:
      | image(imread('HEV_DCDC_System_IMAGE.jpg'));
      | port_label('RConn',1,'Bus+');
      | port_label('RConn',2,'Bus-');
      | port_label('LConn',1,'Batt+');
      | port_label('LConn',2,'Batt-');
      | port_label('RConn',3,'H');
      | text(0.05,0.5,'In');
      | text(0.85,0.5,'Out');
      | %text(0.4,0.8,'Loss');
  " Batt+" : PMIOPort  Tag=PMCPort  Port=1  Side=Left
  " Batt-" : PMIOPort  Tag=PMCPort  Port=2  Side=Left
  " Bus+" : PMIOPort  Tag=PMCPort  Port=3  Side=Right
  " Bus-" : PMIOPort  Tag=PMCPort  Port=4  Side=Right
  H : PMIOPort  Tag=PMCPort  Port=5  Side=Right

== system EVdemo_6/Drive & Motor ==
  note: 1) Only subsystems can be added as variant choices at this level
      | 2) Blocks cannot be connected at this level as connectivity is
      | automatically determined at simulation, based on the active variant
  System Inputs : Inport
  Detailed_Motor : Subsystem  VariantControl=DETAILED_PMSM_CNTRL
      mask Display: image('motordrive.jpg')
  System_Motor : Subsystem  VariantControl=SYSYEM_PMSM_CNTRL
      mask Display: image('simple_motor.jpg')
  + : PMIOPort  Port=1  Side=Left
  R : PMIOPort  Port=2  Side=Right
  - : PMIOPort  Port=3  Side=Left
  H : PMIOPort  Port=4  Side=Left
  Motor_Fdbk : Outport

== system EVdemo_6/Electrical_Partitioin ==
  Controlled Current Source : fl_lib/Electrical/Electrical Sources/Controlled Current Source  i_Log=off  v_Log=off  LocalVarNames=|i|v  LocalVarDescs=|i|v  LocalVarLogging=[0 0]
  Controlled Voltage Source : fl_lib/Electrical/Electrical Sources/Controlled Voltage Source  i_Log=off  v_Log=off  LocalVarNames=|i|v  LocalVarDescs=|i|v  LocalVarLogging=[0 0]
  Current Sensor : fl_lib/Electrical/Electrical Sensors/Current Sensor  i1_Log=off  v1_Log=off  LocalVarNames=|i1|v1  LocalVarDescs=|i1|v1  LocalVarLogging=[0 0]
  GND : fl_lib/Electrical/Electrical Elements/Electrical Reference  i_Log=off  LocalVarNames=|i  LocalVarDescs=|i  LocalVarLogging=0
  "GND " : fl_lib/Electrical/Electrical Elements/Electrical Reference  i_Log=off  LocalVarNames=|i  LocalVarDescs=|i  LocalVarLogging=0
  PS-Simulink Converter1 : nesl_utility/PS-Simulink Converter  PhysicalDomain=network_engine_domain  SubClassName=ps_output  LeftPortType=input  RightPortType=output  PseudoPeriodic=off  Frequencies=[]  Unit=1  AffineConversion=off
  PS-Simulink Converter2 : nesl_utility/PS-Simulink Converter  PhysicalDomain=network_engine_domain  SubClassName=ps_output  LeftPortType=input  RightPortType=output  PseudoPeriodic=off  Frequencies=[]  Unit=1  AffineConversion=off
  Rate Transition1 : RateTransition
  Rate Transition3 : RateTransition
  Simulink-PS Converter : nesl_utility/Simulink-PS Converter  PhysicalDomain=network_engine_domain  SubClassName=ps_input  LeftPortType=input  RightPortType=output  PseudoPeriodic=off  Frequencies=[]  NoiseDistribution=none  NoiseParameters=[]  Unit=1  AffineConversion=off  InputFiltering=off  SimscapeFilterOrder=1  InputFilterTimeConstant=0.001  UdotUserProvided=1
  Simulink-PS Converter1 : nesl_utility/Simulink-PS Converter  PhysicalDomain=network_engine_domain  SubClassName=ps_input  LeftPortType=input  RightPortType=output  PseudoPeriodic=off  Frequencies=[]  NoiseDistribution=none  NoiseParameters=[]  Unit=1  AffineConversion=off  InputFiltering=off  SimscapeFilterOrder=2  InputFilterTimeConstant=1e-3  UdotUserProvided=1
  Voltage Sensor : fl_lib/Electrical/Electrical Sensors/Voltage Sensor  i1_Log=off  v1_Log=off  LocalVarNames=|i1|v1  LocalVarDescs=|i1|v1  LocalVarLogging=[0 0]
  + : PMIOPort  Port=1  Side=Left
  "+ " : PMIOPort  Port=2  Side=Right
  "- " : PMIOPort  Port=3  Side=Right
  - : PMIOPort  Port=4  Side=Left
  wires:
  PS-Simulink Converter1/1 -> Rate Transition3/1
  Rate Transition1/1 -> Simulink-PS Converter1/1
  PS-Simulink Converter2/1 -> Rate Transition1/1
  Rate Transition3/1 -> Simulink-PS Converter/1
  connections:
  "GND "/LConn1 -- Current Sensor/RConn2 -- "- "/RConn1
  -/RConn1 -- GND/LConn1 -- Controlled Current Source/RConn2 -- Voltage Sensor/RConn2
  Voltage Sensor/LConn1 -- +/RConn1 -- Controlled Current Source/LConn1
  Voltage Sensor/RConn1 -- PS-Simulink Converter1/LConn1
  Simulink-PS Converter1/RConn1 -- Controlled Current Source/RConn1
  Current Sensor/LConn1 -- Controlled Voltage Source/RConn2
  Simulink-PS Converter/RConn1 -- Controlled Voltage Source/RConn1
  Controlled Voltage Source/LConn1 -- "+ "/RConn1
  PS-Simulink Converter2/LConn1 -- Current Sensor/RConn1

== system EVdemo_6/Kph Demand ==
  "10-15 mode " : Subsystem  Tag=STV Subsys  LoadFcn=sigbuilder_block('load');  StartFcn=sigbuilder_block('start');  StopFcn=sigbuilder_block('stop');  ClipboardFcn=sigbuilder_block('clipboard');  mask(Sigbuilder block){}
      mask help: Sigbuilder GUI
      mask init:
      | if ~strcmp(get_param(bdroot(gcbh),'SimulationStatus'),'stopped') tuvar = sigbuilder_block('maskInit'); end
      settings: CopyFcn=sigbuilder_block('copy');  DeleteFcn=sigbuilder_block('delete');  ModelCloseFcn=sigbuilder_block('modelClose');  PreSaveFcn=sigbuilder_block('preSave');  PauseFcn=sigbuilder_block('pause')  ContinueFcn=sigbuilder_block('continue')  NameChangeFcn=sigbuilder_block('namechange');  OpenFcn=sigbuilder_block('open',[561.103 179.379 549.931 398.483 ]);  CloseFcn=sigbuilder_block('close');
      mask Display: plot(0,0,100,100,[10,10,40,40,10],[80,20,20,80,80],[40,10],[50,50], [40,27,10],[65,72,56],[40,25,25,10],[28,28,43,43]);
  FTP75 : FromWorkspace  VariableName=[UrbanCycle4.time(ftp75startind:end)-UrbanCycle4.time(ftp75startind) UrbanCycle4.SpdKph(ftp75startind:end)]  SampleTime=0
  FTP75&0260 : FromWorkspace  VariableName=FTP_0260  SampleTime=0
  FTP75&1 : FromWorkspace  VariableName=US06_0260  SampleTime=0
  Ground : Ground
  Multiport Switch : MultiPortSwitch  Inputs=8
  Rate Transition : RateTransition
  Rate Transition1 : RateTransition  OutPortSampleTime=.01
  Rate Transition2 : RateTransition
  Rate Transition3 : RateTransition
  Select Cycle : Constant  Value=Drive_Cycle_Num
  Step : Step  Commented=on  After=100
  US06 : FromWorkspace  VariableName=UrbanCycle6Rep  SampleTime=.01  Interpolate=off  OutputAfterFinalValue=Cyclic repetition
  Urban Cycle 1 : FromWorkspace  VariableName=[UrbanCycle1.time UrbanCycle1.SpdKph]  SampleTime=0
  Urban Cycle 2 : FromWorkspace  VariableName=[UrbanCycle2.time UrbanCycle2.SpdKph]  SampleTime=0
  Urban Cycle 3 : FromWorkspace  VariableName=[UrbanCycle3.time UrbanCycle3.SpdKph]  SampleTime=0
  RefSpd_kph : Outport
  Vehicle_Grade_prct : Outport  Port=2
  wires:
  Urban Cycle 3/1 -> Multiport Switch/4
  Select Cycle/1 -> Multiport Switch/1
  Urban Cycle 2/1 -> Multiport Switch/3
  Urban Cycle 1/1 -> Multiport Switch/2
  Multiport Switch/1 -> RefSpd_kph/1
  FTP75/1 -> Multiport Switch/5
  "10-15 mode "/1(Target speed) -> Multiport Switch/6
  US06/1 -> Rate Transition/1
  Rate Transition/1 -> Multiport Switch/7
  Ground/1 -> Rate Transition1/1
  Rate Transition1/1 -> Vehicle_Grade_prct/1
  FTP75&0260/1 -> Rate Transition2/1
  Rate Transition2/1 -> Multiport Switch/8
  FTP75&1/1 -> Rate Transition3/1
  Rate Transition3/1 -> Multiport Switch/9

== system EVdemo_6/Motor & Power Managment ==
  Operator : Inport  OutDataTypeStr=Bus: Op_Cmds
  Bus : Inport  Port=2  OutDataTypeStr=Bus: Bus_Fdbk
  Motor : Inport  Port=3  OutDataTypeStr=Bus: Motor_Sys_Fdbk
  Veh_Fdbk : Inport  Port=4  OutDataTypeStr=Bus: Veh_Fdbk
  Battery : Inport  Port=5  OutDataTypeStr=Bus: Batt_Fdbk
  EV_Powertrain_Control : ModelReference  ModelNameDialog=EV_Pwr_Manager  SimulationMode=Normal  ModelReferenceVersion=1.285  CopyOfModelName=EV_Pwr_Manager  DefaultDataLogging=on
  Rate Transition{1,4..6,8} (5 alike) : RateTransition
  Unit Delay{1,3..5} (4 alike) : UnitDelay  SampleTime=-1
  ZZZ_Background_Box : Subsystem
      mask Display:
      | % text(0.5, 0.95,'Processor',...
      | %   'HorizontalAlignment', 'Center',...
      | %   'VerticalAlignment', 'Top',...
      | %   'texmode', 'on')
  Control_Status : Outport  OutDataTypeStr=Bus: Cntrl_Status
  Veh_Cmd : Outport  Port=2  OutDataTypeStr=Bus: Veh_Cmds
  Motor_Cmd : Outport  Port=3  OutDataTypeStr=Bus: Motor_Cmds
  wires:
  EV_Powertrain_Control/2 -> Motor_Cmd/1
  EV_Powertrain_Control/1 -> Control_Status/1
  Rate Transition8/1 -> Unit Delay1/1
  Motor/1 -> Rate Transition4/1
  Battery/1 -> Rate Transition5/1
  Operator/1 -> Rate Transition1/1
  Rate Transition5/1 -> Unit Delay4/1
  Rate Transition6/1 -> Unit Delay5/1
  Bus/1 -> Rate Transition6/1
  Veh_Fdbk/1 -> Rate Transition8/1
  Rate Transition4/1 -> Unit Delay3/1
  Rate Transition1/1 -> EV_Powertrain_Control/1
  Unit Delay3/1 -> EV_Powertrain_Control/2
  Unit Delay1/1 -> EV_Powertrain_Control/3
  Unit Delay5/1 -> EV_Powertrain_Control/4
  Unit Delay4/1 -> EV_Powertrain_Control/5
  EV_Powertrain_Control/3 -> Veh_Cmd/1

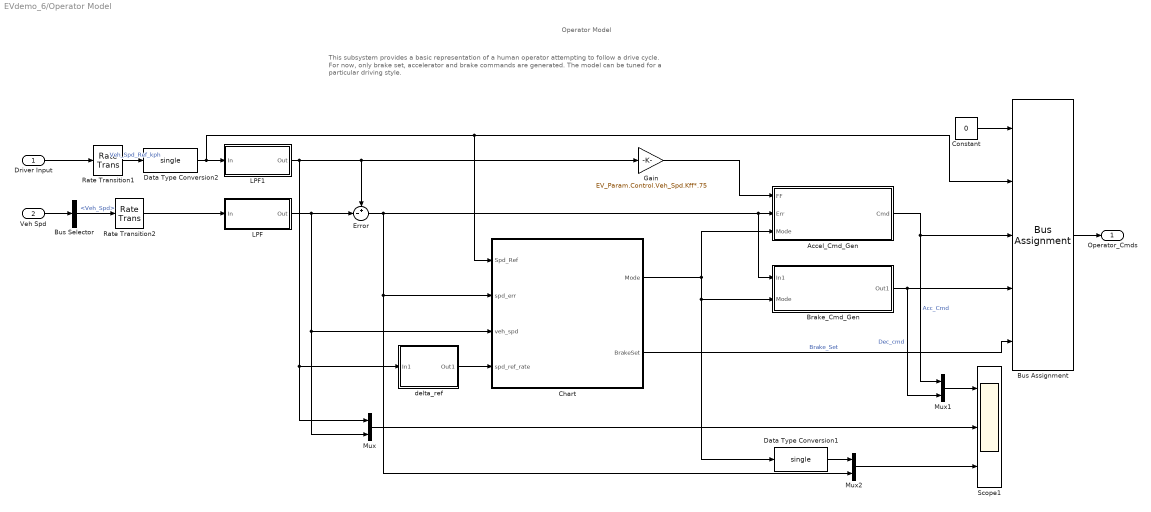
== system EVdemo_6/Operator Model ==
  note: Operator Model
  note: This subsystem provides a basic representation of a human operator attempting to follow a drive cycle. For now, only brake set,
      | accelerator and brake commands are generated. The model can be tuned for a particular driving style.
  Driver Input : Inport
  Veh Spd : Inport  Port=2
  Accel_Cmd_Gen : Subsystem  TreatAsAtomicUnit=on
  Brake_Cmd_Gen : Subsystem  TreatAsAtomicUnit=on
  Bus Assignment : BusAssignment  AssignedSignals=Veh_Spd_Ref,Acc_Cmd,Dec_Cmd,Brake_Set
  Bus Selector : BusSelector  OutputSignals=Veh_Spd
  Chart : Stateflow chart  TreatAsAtomicUnit=on
  Constant : Constant  Value=0  OutDataTypeStr=Bus: Op_Cmds  SampleTime=-1
  Data Type Conversion1 : DataTypeConversion  OutDataTypeStr=single
  Data Type Conversion2 : DataTypeConversion  OutDataTypeStr=single
  Error : Sum  Inputs=+-|  OutDataTypeStr=single
  Gain : Gain  Gain=EV_Param.Control.Veh_Spd.Kff*.75  ParamDataTypeStr=Inherit: Inherit from 'Gain'
  LPF : Subsystem  mask{w=30*pi*2}
      mask prompts: w "w(rad/s)"
      mask Display:
      | fprintf('LPF')
      | port_label('output', 1, 'out')
      | port_label('input', 1, 'in')
  LPF1 : Subsystem  mask{w=10*pi*2}
      mask prompts: w "w(rad/s)"
      mask Display:
      | fprintf('LPF')
      | port_label('output', 1, 'out')
      | port_label('input', 1, 'in')
  Mux : Mux  Inputs=2
  Mux1 : Mux  Inputs=2
  Mux2 : Mux  Inputs=2
  Rate Transition1 : RateTransition  OutPortSampleTime=.01
  Rate Transition2 : RateTransition  OutPortSampleTime=.01
  Scope1 : Scope  NumInputPorts=3
      settings: YMin=-1~-10~-20  YMax=2.5~130~130  SaveName=ScopeData19
  delta_ref : Subsystem
  Operator_Cmds : Outport
  wires:
  Bus Assignment/1 -> Operator_Cmds/1
  Veh Spd/1 -> Bus Selector/1
  Accel_Cmd_Gen/1(Cmd) -> Bus Assignment/3, Mux1/1  "Acc_Cmd"
  Rate Transition1/1 -> Data Type Conversion2/1  "Veh_Spd_Ref_kph"
  Gain/1 -> Accel_Cmd_Gen/1(FF)
  LPF1/1(Out) -> Gain/1, Error/1, Mux/1, delta_ref/1(In1)
  Rate Transition2/1 -> LPF/1(In)
  Bus Selector/1 -> Rate Transition2/1  "<Veh_Spd>"
  Error/1 -> Mux2/2, Chart/2(spd_err), Brake_Cmd_Gen/1(In1), Accel_Cmd_Gen/2(Err)
  Chart/1(Mode) -> Accel_Cmd_Gen/3(Mode), Data Type Conversion1/1, Brake_Cmd_Gen/2(Mode)
  Mux/1 -> Scope1/2
  Driver Input/1 -> Rate Transition1/1
  LPF/1(Out) -> Mux/2, Chart/3(veh_spd), Error/2
  Brake_Cmd_Gen/1(Out1) -> Bus Assignment/4, Mux1/2  "Dec_cmd"
  Mux1/1 -> Scope1/1
  Chart/2(BrakeSet) -> Bus Assignment/5  "Brake_Set"
  Mux2/1 -> Scope1/3
  Data Type Conversion1/1 -> Mux2/1
  delta_ref/1(Out1) -> Chart/4(spd_ref_rate)
  Constant/1 -> Bus Assignment/1
  Data Type Conversion2/1 -> Chart/1(Spd_Ref), Bus Assignment/2, LPF1/1(In)
